simulink model "controladorpruebaio"  (R2025a)
settings: Solver=FixedStepAuto  StartTime=0.0  StopTime=inf  FixedStep=0.015  RelTol=1e-3  EnableMultiTasking=on
libraries: px4Peripheralslib x1, px4uORBlib x1, px4Sensorslib x1
settings Model: PacingRate=0.790000  ExtModeTrigDuration=10  Creator=The MathWorks, Inc.  LastModifiedBy=aero
settings SolverCC: AlgebraicLoopSolver=TrustRegion  PositivePriorityOrder=on  AutoInsertRateTranBlk=on  MaxZcPerStep=1.0
settings OptimizationCC: EnhancedBackFolding=on  PassReuseOutputArgsAs=Individual arguments  MaxStackSize=64  OptimizeBlockOrder=speed  DifferentSizesBufferReuse=on  OptimizationCustomize=off  EfficientTunableParamExpr=on
settings DebuggingCC: ParameterPrecisionLossMsg=none  ParameterTunabilityLossMsg=error  UnconnectedInputMsg=warning  UnconnectedOutputMsg=warning  UnconnectedLineMsg=warning  SubsystemReferenceDiagnosticForUnitTest=warning  ArithmeticOperatorsInVariantConditions=warning
settings HardwareCC: ProdBitPerPointer=32.0  ProdBitPerSizeT=32.0  ProdBitPerPtrDiffT=32.0  ProdLargestAtomicInteger=Long  ProdLargestAtomicFloat=Double  ProdWordSize=32.0  ProdLongLongMode=on  ProdHWDeviceType=ARM Compatible->ARM Cortex
settings ModelReferenceCC: EnableRefExpFcnMdlSchedulingChecks=on
settings SFSimCC: MATLABDynamicMemAlloc=off  SimTargetLang=C++  SimDLTargetLibrary=mkl-dnn
settings RTWCC: SystemTargetFile=ert.tlc  HardwareBoard=PX4 Pixhawk 6c  TLCOptions="-aInlineSetEventsForThisBaseRateFcn=TLC_FALSE -aSuppressMultiTaskScheduler=TLC_FALSE  -aRateBasedStepFcn=0"  TemplateMakefile=ert_default_tmf  GenerateReport=on  Toolchain=GNU Tools for PX4 Autopilots  IncludeHyperlinkInReport=on  LaunchReport=on  TargetLang=C++  GenerateTraceInfo=on  GenerateTraceReport=on  GenerateTraceReportSl=on  GenerateTraceReportSf=on  GenerateTraceReportEml=on  GPUComputeCapability=3.5  DLArmComputeVersion=19.05  Description=Embedded Coder
settings CodeAppCC: ForceParamTrailComments=on  IgnoreCustomStorageClasses=off  OperatorAnnotations=on  SimulinkDataObjDesc=on  SFDataObjDesc=on  InsertBlockDesc=on
settings ERTTargetCC: ExtModeTransport=3.0  ExtModeStaticAllocSize=1024.0  InlinedParameterPlacement=Hierarchical

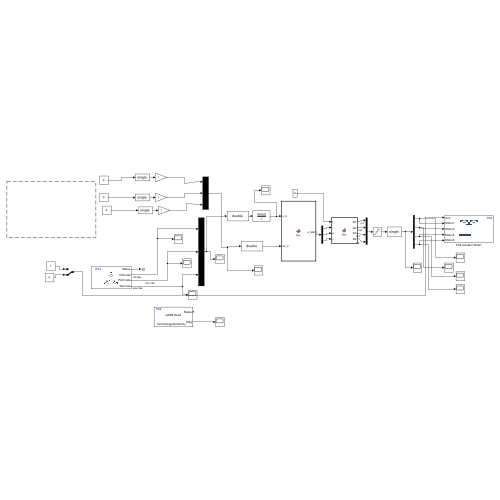
[thumbnail: Simulink's stored preview of the top-level diagram]
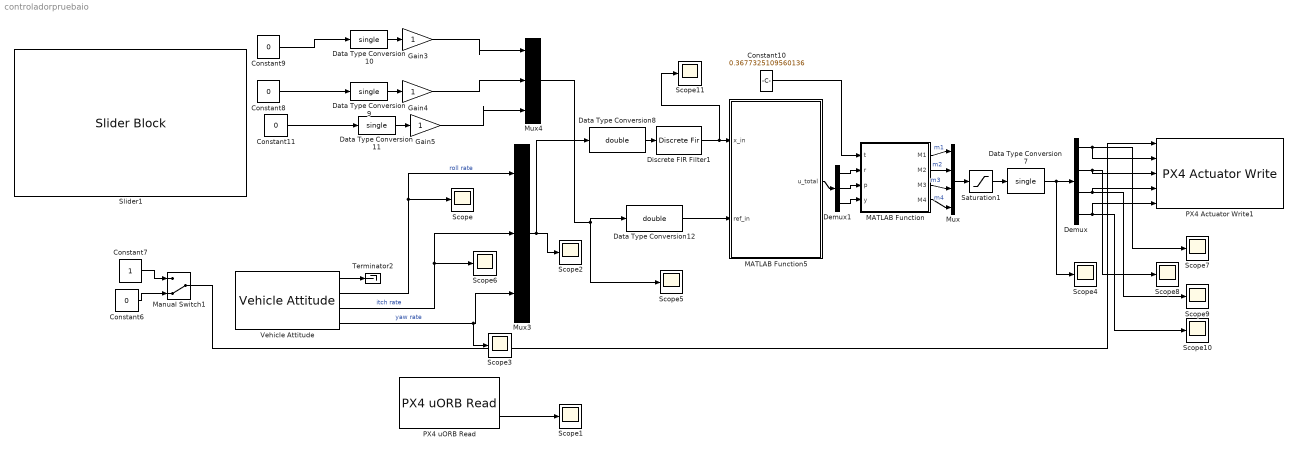
== system controladorpruebaio ==
  Constant10 : Constant  Value=0.3677325109560136
  Constant11 : Constant  Value=0
  Constant6 : Constant  Value=0  OutDataTypeStr=boolean
  Constant7 : Constant  OutDataTypeStr=boolean
  Constant8 : Constant  Value=0
  Constant9 : Constant  Value=0
  Data Type Conversion{7,9..11} (4 alike) : DataTypeConversion  OutDataTypeStr=single  SaturateOnIntegerOverflow=off  RndMeth=Floor
  Data Type Conversion12 : DataTypeConversion  OutDataTypeStr=double  SaturateOnIntegerOverflow=off  RndMeth=Floor  LockScale=on
  Data Type Conversion8 : DataTypeConversion  OutDataTypeStr=double  SaturateOnIntegerOverflow=off  RndMeth=Floor  LockScale=on
  Demux : Demux
  Demux1 : Demux  Outputs=3
  Discrete FIR Filter1 : DiscreteFir  Coefficients=[0.2 0.2 0.2 0.2 0.2]
  Gain3 : Gain
  Gain4 : Gain
  Gain5 : Gain
  MATLAB Function : MATLAB Function  TreatAsAtomicUnit=on
  MATLAB Function5 : MATLAB Function  TreatAsAtomicUnit=on
  Manual Switch1 : ManualSwitch  CurrentSetting=0
  Mux : Mux
  Mux3 : Mux  Inputs=3
  Mux4 : Mux  Inputs=3
  PX4 Actuator Write1 : px4Peripheralslib/PX4 Actuator Write  Motor1Enable=on  Motor2Enable=on  Motor3Enable=on  Motor4Enable=on  Motor5Enable=off  Motor6Enable=off  Motor7Enable=off  Motor8Enable=off  Motor9Enable=off  Motor10Enable=off  Motor11Enable=off  Motor12Enable=off  IsMotorArray=off  Servo1Enable=off  Servo2Enable=off  Servo3Enable=off  Servo4Enable=off  Servo5Enable=off  Servo6Enable=off  Servo7Enable=off  Servo8Enable=off  IsServoArray=off
  PX4 uORB Read : px4uORBlib/PX4 uORB Read  uORBTopic=VehicleAngularVelocity  selectInstance=vehicle_angular_velocity  SampleTime=0.015  BlockingMode=off  BlockTimeout=1e-3
  Saturation1 : Saturate  UpperLimit=1  LowerLimit=0
  Scope{,1..11} (12 alike) : Scope
      Scope settings: ActiveDisplayYMinimum=-0.37485260516405106  ActiveDisplayYMaximum=0.45409966260194778
      Scope1 settings: ActiveDisplayYMinimum=-0.699282243847847  ActiveDisplayYMaximum=1.0211267024278641  DataLoggingVariableName=ScopeData2
      Scope10 settings: ActiveDisplayYMinimum=0.36480339616537094  ActiveDisplayYMaximum=0.37054816633462906  DataLoggingVariableName=ScopeData10
      Scope11 settings: DataLoggingVariableName=ScopeData11
      Scope2 settings: ActiveDisplayYMinimum=-0.007830842916480887  ActiveDisplayYMaximum=0.011785188651862866
      Scope3 settings: ActiveDisplayYMinimum=-0.701383207950559  ActiveDisplayYMaximum=0.652295516106815  DataLoggingVariableName=ScopeData3
      Scope4 settings: ActiveDisplayYMinimum=-1.5029836862276127  ActiveDisplayYMaximum=1.9132041073394161  DataLoggingVariableName=ScopeData4
      Scope5 settings: ActiveDisplayYMinimum=-1  ActiveDisplayYMaximum=1  DataLoggingVariableName=ScopeData5
      Scope6 settings: ActiveDisplayYMinimum=-0.31608365406560018  ActiveDisplayYMaximum=0.26270581930166403  DataLoggingVariableName=ScopeData6
      Scope7 settings: ActiveDisplayYMinimum=-0.079447194933891283  ActiveDisplayYMaximum=0.71502475440502167  DataLoggingVariableName=ScopeData7
      Scope8 settings: ActiveDisplayYMinimum=-0.07054468989372252  ActiveDisplayYMaximum=0.63490220904350281  DataLoggingVariableName=ScopeData8
      Scope9 settings: ActiveDisplayYMinimum=-0.03693903284147379  ActiveDisplayYMaximum=0.83852717699483037  DataLoggingVariableName=ScopeData9
  Slider1 : SliderBlock  ScaleMax=0.6
  Terminator2 : Terminator
  Vehicle Attitude : px4Sensorslib/Vehicle Attitude  rollRate=on  pitchRate=on  yawRate=on  quaternion=off  uorbTimeStamp=off  BlockingMode=off  BlockTimeout=0.001  sampleTime=0.015
  wires:
  Demux/4 -> Scope10/1, PX4 Actuator Write1/5
  Vehicle Attitude/3 -> Mux3/2, Scope6/1  "itch rate"
  Data Type Conversion8/1 -> Discrete FIR Filter1/1
  Data Type Conversion7/1 -> Scope4/1, Demux/1
  Constant6/1 -> Manual Switch1/2
  Constant9/1 -> Data Type Conversion10/1
  Vehicle Attitude/4 -> Scope3/1, Mux3/3  "yaw rate"
  MATLAB Function/2(M2) -> Mux/2  "m2"
  MATLAB Function/3(M3) -> Mux/3  "m3"
  Gain4/1 -> Mux4/2
  Demux/3 -> Scope9/1, PX4 Actuator Write1/4
  Constant10/1 -> MATLAB Function/1(t)
  Gain5/1 -> Mux4/3
  Mux4/1 -> Scope5/1, Data Type Conversion12/1
  PX4 uORB Read/2 -> Scope1/1
  Data Type Conversion12/1 -> MATLAB Function5/2(ref_in)
  Vehicle Attitude/1 -> Terminator2/1
  Gain3/1 -> Mux4/1
  Saturation1/1 -> Data Type Conversion7/1
  Constant7/1 -> Manual Switch1/1
  Demux1/2 -> MATLAB Function/3(p)
  Data Type Conversion9/1 -> Gain4/1
  Demux1/3 -> MATLAB Function/4(y)
  Data Type Conversion10/1 -> Gain3/1
  Demux1/1 -> MATLAB Function/2(r)
  Demux/1 -> Scope7/1, PX4 Actuator Write1/2
  Demux/2 -> Scope8/1, PX4 Actuator Write1/3
  Mux/1 -> Saturation1/1
  Mux3/1 -> Scope2/1, Data Type Conversion8/1
  MATLAB Function5/1(u_total) -> Demux1/1
  Vehicle Attitude/2 -> Scope/1, Mux3/1  "roll rate"
  Data Type Conversion11/1 -> Gain5/1
  Constant8/1 -> Data Type Conversion9/1
  Constant11/1 -> Data Type Conversion11/1
  MATLAB Function/4(M4) -> Mux/4  "m4"
  Manual Switch1/1 -> PX4 Actuator Write1/1
  MATLAB Function/1(M1) -> Mux/1  "m1"
  Discrete FIR Filter1/1 -> Scope11/1, MATLAB Function5/1(x_in)

== matlab function controladorpruebaio/MATLAB Function ==
  data: t input; M1 output; r input; p input; y input; M2 output; M3 output; M4 output
function [M1,M2,M3,M4] = fcn(t, r, p, y)
% t: thrust
% r: roll
% p: pitch
% y: yaw

M1 = t - r + p + y;
M2 = t + r - p + y;
M3 = t + r + p - y;
M4 = t - r - p - y;

== matlab function controladorpruebaio/MATLAB Function5 ==
  data: x_in input; u_total output; ref_in input
function u_total = fcn(x_in, ref_in)
%#codegen

% --- CONFIGURACIÓN ESTÁTICA ---
persistent A B Phi F_f H  options lb ub Q_big
    
if isempty(A)
    % 1. Matrices del sistema
        A = [1.333650695949998	-1.668714910244021	5.632342547392557;
            1.220605709316355	-1.768083035175748	2.980769476932811;
            0.324324414735769	-0.426047177599778	-0.281734621621188];
        B = [-2.122185994762327	-1.353681217245696	-1.462094492977615;
            -1.013280130692134	-1.854604300287162 -0.351287697129404;
            0.578625448174987	-0.128607817414752	0.510736009980700];

        
    % Pre-dimensionado total (N=6, nx=3, nu=3 -> 18)
    F_mat = zeros(18, 3);
    Phi_mat = zeros(18, 18);
    Q_big_mat = zeros(18, 18);
    R_big_mat = zeros(18, 18);
    
    Q_inst = eye(3) * 1; 
    R_inst = diag([40 40 40]); 
        
    % Llenado de matrices con índices fijos para el compilador
    for i = 1:6
        row = (i-1)*3 + (1:3); % Esto es aceptado por Coder
        F_mat(row, :) = A^i;
        Q_big_mat(row, row) = Q_inst;
        R_big_mat(row, row) = R_inst;
        
        for j = 1:i
            col = (j-1)*3 + (1:3);
            Phi_mat(row, col) = A^(i-j) * B;
        end
    end
        
    H = 2 * (Phi_mat' * Q_big_mat * Phi_mat + R_big_mat);
    F_f = 2 * Phi_mat' * Q_big_mat * F_mat;
    Phi = Phi_mat; 
    Q_big = Q_big_mat;
        

           
    options = optimoptions('quadprog', 'Algorithm', 'active-set', 'Display', 'off');
    
    % Definición directa de límites
    lb = -1 * ones(18, 1); 
    ub =  1 * ones(18, 1);
end

% --- PROCESAMIENTO ---
x = double(x_in(:));
ref_vec = double(ref_in(:));


% --- LÓGICA MPC ---
U0 = zeros(18, 1); 
Ref_seq = repmat(ref_vec, 6, 1);
f = F_f * x - (2 * Phi' * Q_big * Ref_seq);
    
[U_sol, ~, exitflag] = quadprog(H, f, [], [], [], [], lb, ub, U0, options);
    
u = zeros(3,1);
if exitflag > 0
    u = U_sol(1:3);
end
    
% Mezcla final
u_total = [u(1); u(2); u(3)];
